simulink model "ESP32_CONTROL_SYSTEM"  (R2024a)
settings: Solver=FixedStepAuto  StartTime=0.0  StopTime=inf  FixedStep=0.05  RelTol=1e-3
values from neighbouring files (symbols this model uses):
  Beta1 = 3*Omega_o    (= 150)    [ESP32_ANALOG_READ_VAR.m]
  Beta2 = 3*(Omega_o^2)    (= 7500)    [ESP32_ANALOG_READ_VAR.m]
  Beta3 = (Omega_o^3)    (= 125000)    [ESP32_ANALOG_READ_VAR.m]
  Desire_Max = 255    [ESP32_ANALOG_READ_VAR.m]
  Desire_Min = 0    [ESP32_ANALOG_READ_VAR.m]
  Direction_Pin = 0    [ESP32_ANALOG_READ_VAR.m]
  EN_Pin = 1    [ESP32_ANALOG_READ_VAR.m]
  J_aet = 0.0035    [ESP32_ANALOG_READ_VAR.m]
  Kd = 1    [ESP32_ANALOG_READ_VAR.m]
  Ki = 2    [ESP32_ANALOG_READ_VAR.m]
  Kp = 3    [ESP32_ANALOG_READ_VAR.m]
  omga_c = 2    [ESP32_ANALOG_READ_VAR.m]
  roa = 0.24    [ESP32_ANALOG_READ_VAR.m]
libraries: arduinolib x6, simulink_extras x5, simulink x1
(part 1 of 3)
settings Model: ExtModeTrigDuration=2  Creator=obell  LastModifiedBy=Banana444
settings SolverCC: AutoInsertRateTranBlk=on
settings OptimizationCC: EnhancedBackFolding=on  PassReuseOutputArgsAs=Individual arguments  ZeroExternalMemoryAtStartup=off  ZeroInternalMemoryAtStartup=off  MaxStackSize=64  OptimizeBlockOrder=speed  DifferentSizesBufferReuse=on  OptimizationCustomize=off  EfficientTunableParamExpr=on
settings DebuggingCC: ParameterTunabilityLossMsg=error
settings HardwareCC: ProdBitPerPointer=32  ProdBitPerSizeT=32  ProdBitPerPtrDiffT=32  ProdLargestAtomicInteger=Long  ProdLargestAtomicFloat=Double  ProdWordSize=32  ProdLongLongMode=on  ProdHWDeviceType=ARM Compatible->ARM Cortex
settings SFSimCC: MATLABDynamicMemAlloc=off
settings RTWCC: Description=Embedded Coder  SystemTargetFile=ert.tlc  HardwareBoard=ESP32-WROOM(Arduino Compatible)  TLCOptions="-aInlineSetEventsForThisBaseRateFcn=TLC_FALSE -aSuppressMultiTaskScheduler=TLC_FALSE  -aRateBasedStepFcn=0"  TemplateMakefile=ert_default_tmf  Toolchain=ESP32
settings CodeAppCC: ForceParamTrailComments=on  IgnoreCustomStorageClasses=off  OperatorAnnotations=on  SimulinkDataObjDesc=on  SFDataObjDesc=on  InsertBlockDesc=on
settings ERTTargetCC: SupportContinuousTime=on  SupportVariableSizeSignals=on  ExtModeTransport=3  ExtModeStaticAlloc=on  ExtModeAutomaticAllocSize=off  ExtModeStaticAllocSize=65536  ExtModeMexFile=ext_xcp  ExtModeIntrfLevel=Level2 - Open

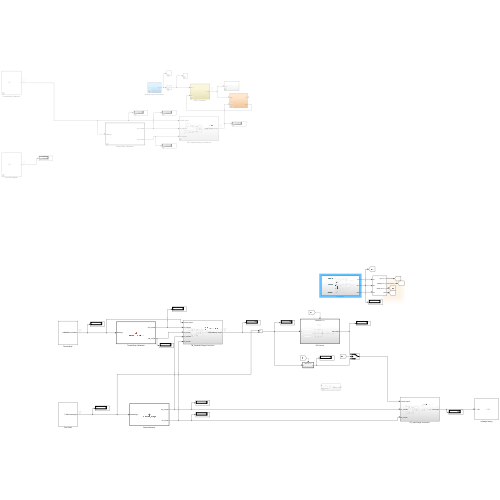
[thumbnail: Simulink's stored preview of the top-level diagram]
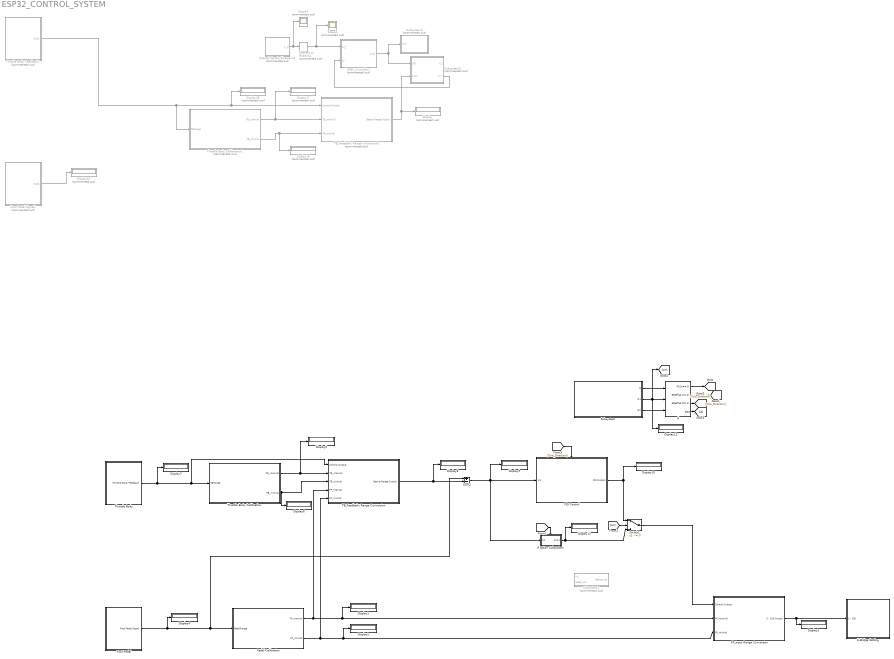
== system ESP32_CONTROL_SYSTEM ==
  Degrees to Radians2 : simulink_extras/Transformations/Degrees to Radians  Commented=on
  Desired signals_Sinewave1 : Subsystem  Commented=on
  Display{,16..17,25,28} (5 alike) : Display  Commented=on
      Display25 settings: Decimation=2
      Display28 settings: Decimation=2
  Display{1..12} (12 alike) : Display
      settings: Decimation=2
  FP_Input Range Conversion : Subsystem
  Foot Pedal : Subsystem
      mask Display: image('Padle-removebg-preview.png');
  Foot Pedal Signal1 : Subsystem  Commented=on
      mask Display: image('Padle-removebg-preview.png');
  Goto3 : Goto
  H-Bridge Setting : Subsystem
      mask Display: image('H-Bridge.JPG');
  If : If  NumInputs=3  IfExpression=u1 == 1  ElseIfExpressions=u2 == 1, u3 == 1
  If Action Subsystem : Subsystem  TreatAsAtomicUnit=on
  PID Control : Subsystem
  Pedal Calibration : MATLAB Function  TreatAsAtomicUnit=on
  SFBC_Controller1 : Subsystem  Commented=on
  Scope2 : Scope  Commented=on
  Scope3 : Scope  Commented=on
  Subsystem : Subsystem
  Subsystem1 : Subsystem  Commented=on
  Subsystem4 : Subsystem  Commented=on
  Subsystem5 : Subsystem  Commented=on
  Sum2 : Sum  Inputs=+-
  Switch1 : Switch  Criteria=u2 ~= 0  Threshold=1  SaturateOnIntegerOverflow=off  InputSameDT=off
  TB_Feedbakc Range Conversion : Subsystem
  TB_Feedbakc Range Conversion3 : Subsystem  Commented=on
  "Throttle Body " : Subsystem
      mask Display: image('electronic-throttle-body.png');
  Throttle Body Callibration : MATLAB Function  TreatAsAtomicUnit=on
  Throttle Body Callibration1 : MATLAB Function  Commented=on  TreatAsAtomicUnit=on
  Throttle Body Feedback1 : Subsystem  Commented=on
      mask Display: image('electronic-throttle-body.png');
  wires:
  Pedal Calibration/2(FP_minVal) -> TB_Feedbakc Range Conversion/5(FP_minVal), Display2/1, FP_Input Range Conversion/3(FP_minVal)
  Throttle Body Callibration/1(TB_maxVal) -> Display5/1, TB_Feedbakc Range Conversion/2(TB_maxVal)
  Pedal Calibration/1(FP_maxVal) -> Display1/1, FP_Input Range Conversion/2(FP_maxVal), TB_Feedbakc Range Conversion/4(FP_maxVal)
  FP_Input Range Conversion/1(0 - 100 Output) -> H-Bridge Setting/1(1 - 100), Display3/1
  Subsystem/1(Q) -> If/1
  Subsystem/3(Q2) -> If/3
  Subsystem/2(Q1) -> Display11/1, [on], If/2
  If/1 -> [Regular]
  If/2 -> [One_Direction]
  If/3 -> [Two_Direction]
  If/4 -> Goto3/1
  [Regular] -> If Action Subsystem/Action
  PID Control/1(PID Output) -> Switch1/1, Display10/1
  If Action Subsystem/1(Out1) -> Switch1/3, Display12/1
  [One_Direction] -> PID Control/Action
  Switch1/1 -> FP_Input Range Conversion/1(Control Output)
  Sum2/1 -> If Action Subsystem/1(In1), PID Control/1(In1), Display9/1
  [on] -> Switch1/2
  TB_Feedbakc Range Conversion/1(" Desire Range Output") -> Sum2/2, Display8/1
  "Throttle Body "/1(Throttle Body Feedback) -> Display7/1, Throttle Body Callibration/1(TBRange), TB_Feedbakc Range Conversion/1(Control Output)
  Foot Pedal/1(Foot Pedal Signal) -> Display4/1, Sum2/1, Pedal Calibration/1(PedalRange)
  Throttle Body Callibration/2(TB_minVal) -> TB_Feedbakc Range Conversion/3(TB_minVal), Display6/1
  Desired signals_Sinewave1/1(xi_d) -> Scope3/1, Degrees to Radians2/1
  Degrees to Radians2/1 -> Scope2/1, SFBC_Controller1/1(Xd_i)
  Foot Pedal Signal1/1(Out1) -> Display25/1
  Throttle Body Feedback1/1(Out1) -> Throttle Body Callibration1/1(TBRange), Display28/1, TB_Feedbakc Range Conversion3/1(Control Output)
  SFBC_Controller1/1(U (t)) -> Subsystem5/1(U(t)), Subsystem4/1(U(t))
  TB_Feedbakc Range Conversion3/1(" Desire Range Output") -> Display/1, Subsystem5/2(X1(t))
  Subsystem5/2(Xi^) -> SFBC_Controller1/2(Xi^)
  Throttle Body Callibration1/1(TB_maxVal) -> Display17/1, TB_Feedbakc Range Conversion3/2(TB_maxVal)
  Throttle Body Callibration1/2(TB_minVal) -> Display16/1, TB_Feedbakc Range Conversion3/3(TB_minVal)

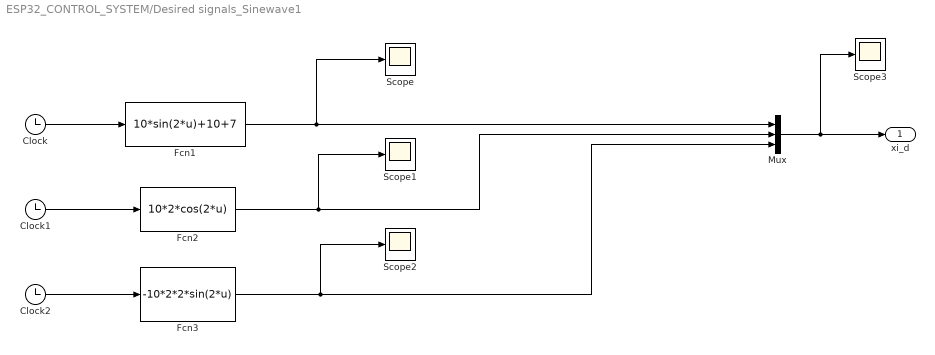
== system ESP32_CONTROL_SYSTEM/Desired signals_Sinewave1 ==
  Clock : Clock
  Clock1 : Clock
  Clock2 : Clock
  Fcn1 : Fcn  Expr=10*sin(2*u)+10+7
  Fcn2 : Fcn  Expr=10*2*cos(2*u)
  Fcn3 : Fcn  Expr=-10*2*2*sin(2*u)
  Mux : Mux  Inputs=3
  Scope{,1..3} (4 alike) : Scope
  xi_d : Outport
  wires:
  Fcn1/1 -> Scope/1, Mux/1
  Fcn2/1 -> Scope1/1, Mux/2
  Fcn3/1 -> Scope2/1, Mux/3
  Mux/1 -> Scope3/1, xi_d/1
  Clock/1 -> Fcn1/1
  Clock1/1 -> Fcn2/1
  Clock2/1 -> Fcn3/1

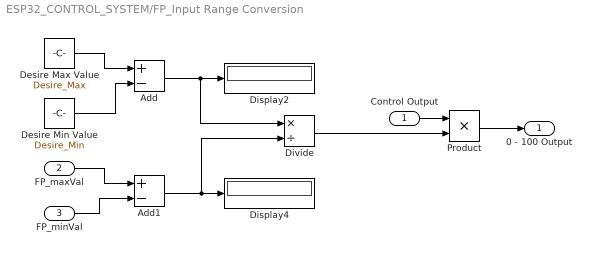
== system ESP32_CONTROL_SYSTEM/FP_Input Range Conversion ==
  Control Output : Inport
  FP_maxVal : Inport  Port=2
  FP_minVal : Inport  Port=3
  Add : Sum  Inputs=+-
  Add1 : Sum  Inputs=+-
  Desire Max Value : Constant  Value=Desire_Max
  Desire Min Value : Constant  Value=Desire_Min
  Display2 : Display
  Display4 : Display
  Divide : Product  Inputs=*/
  Product : Product
  0 - 100 Output : Outport
  wires:
  Add/1 -> Divide/1, Display2/1
  FP_minVal/1 -> Add1/2
  Add1/1 -> Divide/2, Display4/1
  Desire Max Value/1 -> Add/1
  Divide/1 -> Product/2
  Desire Min Value/1 -> Add/2
  Control Output/1 -> Product/1
  Product/1 -> 0 - 100 Output/1
  FP_maxVal/1 -> Add1/1

== system ESP32_CONTROL_SYSTEM/Foot Pedal ==
  ESP23_ANALOG_READ_DDAppGeneratedBlock1 : MATLABSystem  System=ESP32_ANALOG_READ  PIN=int8( 34 )  SampleTime=-1
      mask Type: ESP32_ANALOG_READ
      mask Display:
      | color('white');plot([100,100,100,100]*1,[100,100,100,100]*1);plot([100,100,100,100]*0,[100,100,100,100]*0);color('blue');text(38, 92, 'IO Device Builder','horizontalAlignment', 'right');
      | color('black');text(52,50,' ESP32_ANALOG_READ','horizontalAlignment','center');
      | port_label('output',1,'V');
  Foot Pedal Signal : Outport
  wires:
  ESP23_ANALOG_READ_DDAppGeneratedBlock1/1 -> Foot Pedal Signal/1

== system ESP32_CONTROL_SYSTEM/Foot Pedal Signal1 ==
  ESP23_ANALOG_READ_DDAppGeneratedBlock1 : MATLABSystem  System=ESP32_ANALOG_READ  PIN=int8( 34 )  SampleTime=-1
      mask Type: ESP32_ANALOG_READ
      mask Display:
      | color('white');plot([100,100,100,100]*1,[100,100,100,100]*1);plot([100,100,100,100]*0,[100,100,100,100]*0);color('blue');text(38, 92, 'IO Device Builder','horizontalAlignment', 'right');
      | color('black');text(52,50,' ESP32_ANALOG_READ','horizontalAlignment','center');
      | port_label('output',1,'V');
  Out1 : Outport
  wires:
  ESP23_ANALOG_READ_DDAppGeneratedBlock1/1 -> Out1/1

== system ESP32_CONTROL_SYSTEM/H-Bridge Setting ==
  1 - 100 : Inport
  Digital Output : arduinolib/Digital Output  pinNumber=4  Direction=output  blockPlatform=arduino
  Digital Output1 : arduinolib/Digital Output  pinNumber=0  Direction=output  blockPlatform=arduino
  Direction Pin : Constant  Value=Direction_Pin
  Display3 : Display
  Display4 : Display
  Enable Pin : Constant  Value=EN_Pin
  PWM : arduinolib/PWM  pinNumber=2  frequencyType=Specify  desiredFrequency=19000  achievableFrequency=19000
  wires:
  Enable Pin/1 -> Display4/1, Digital Output/1
  1 - 100/1 -> PWM/1
  Direction Pin/1 -> Display3/1, Digital Output1/1

== system ESP32_CONTROL_SYSTEM/If Action Subsystem ==
  In1 : Inport
  Action Port : ActionPort  ActionPortLabel=if(u1 == 1)
  Out1 : Outport
  wires:
  In1/1 -> Out1/1

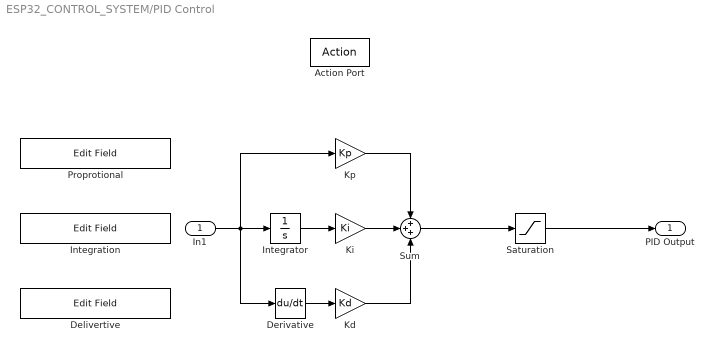
== system ESP32_CONTROL_SYSTEM/PID Control ==
  In1 : Inport
  Action Port : ActionPort  ActionPortLabel=elseif(u2 == 1)
  Delivertive : EditField  LabelPosition=Hide  ShowInitialText=on  Alignment=Center
  Derivative : Derivative
  Integration : EditField  LabelPosition=Hide  ShowInitialText=on  Alignment=Center
  Integrator : Integrator
  Kd : Gain  Gain=Kd
  Ki : Gain  Gain=Ki
  Kp : Gain  Gain=Kp
  Proprotional : EditField  LabelPosition=Hide  ShowInitialText=on  Alignment=Center
  Saturation : Saturate  UpperLimit=3  LowerLimit=0
  Sum : Sum  Inputs=+++
  PID Output : Outport
  wires:
  In1/1 -> Integrator/1, Derivative/1, Kp/1
  Integrator/1 -> Ki/1
  Kp/1 -> Sum/1
  Sum/1 -> Saturation/1
  Ki/1 -> Sum/2
  Derivative/1 -> Kd/1
  Kd/1 -> Sum/3
  Saturation/1 -> PID Output/1

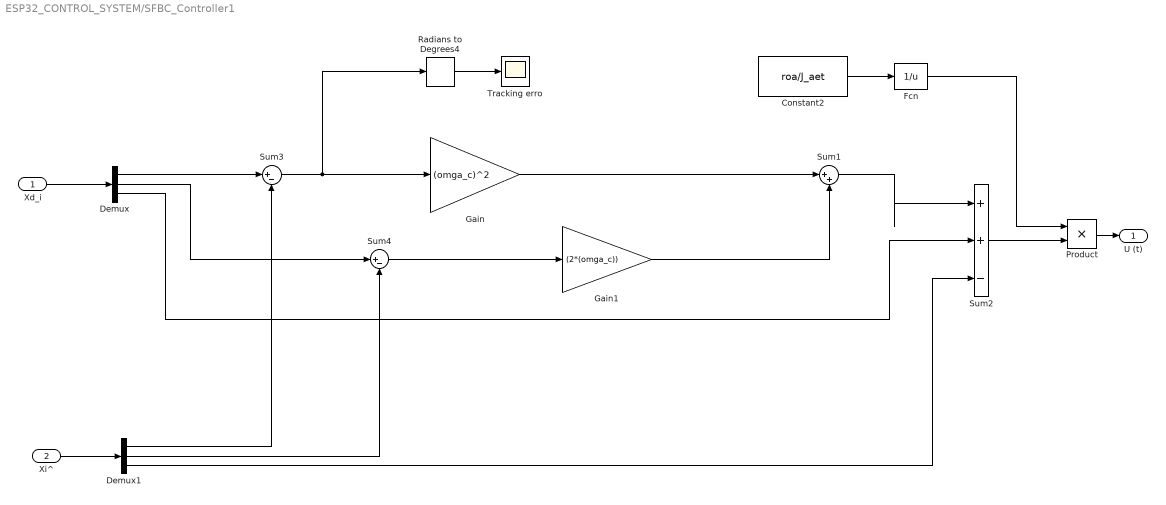
== system ESP32_CONTROL_SYSTEM/SFBC_Controller1 ==
  Xd_i : Inport
  Xi^ : Inport  Port=2
  Constant2 : Constant  Value=roa/J_aet
  Demux : Demux  Outputs=3
  Demux1 : Demux  Outputs=3
  Fcn : Fcn  Expr=1/u
  Gain : Gain  Gain=(omga_c)^2
  Gain1 : Gain  Gain=(2*(omga_c))
  Product : Product  RndMeth=Zero
  Radians to Degrees4 : simulink_extras/Transformations/Radians to Degrees
  Sum1 : Sum  Inputs=|++
  Sum2 : Sum  Inputs=|++-
  Sum3 : Sum  Inputs=|+-
  Sum4 : Sum  Inputs=|+-
  Tracking erro : Scope
  U (t) : Outport
  wires:
  Gain/1 -> Sum1/1
  Gain1/1 -> Sum1/2
  Sum1/1 -> Sum2/1
  Constant2/1 -> Fcn/1
  Fcn/1 -> Product/1
  Sum2/1 -> Product/2
  Demux1/3 -> Sum2/3
  Product/1 -> U (t)/1
  Demux/3 -> Sum2/2
  Sum4/1 -> Gain1/1
  Xd_i/1 -> Demux/1
  Demux/1 -> Sum3/1
  Xi^/1 -> Demux1/1
  Demux1/1 -> Sum3/2
  Demux/2 -> Sum4/1
  Demux1/2 -> Sum4/2
  Sum3/1 -> Radians to Degrees4/1, Gain/1
  Radians to Degrees4/1 -> Tracking erro/1
